simulink model "PMSM_DTC_Traditional_Control"  (R2022b)
settings: Solver=ode23tb  StartTime=0.0  StopTime=0.4  RelTol=1e-4
libraries: spsDCVoltageSourceLib x1, spsGroundLib x1, slpidlib x1, spsPermanentMagnetSynchronousMachineLib x1, spsThreePhaseVIMeasurementLib x1, spsTwoLevelConverterLib x1, spspowerguiLib x1
settings Model: Creator=31904  LastModifiedBy=31904
settings SolverCC: ZeroCrossAlgorithm=Adaptive
settings DebuggingCC: IgnoredZcDiagnostic=none

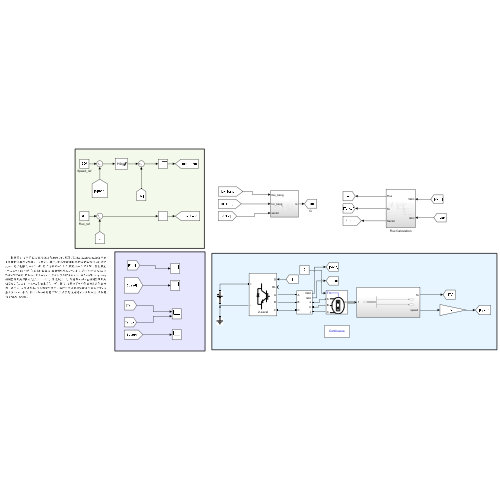
[thumbnail: Simulink's stored preview of the top-level diagram]
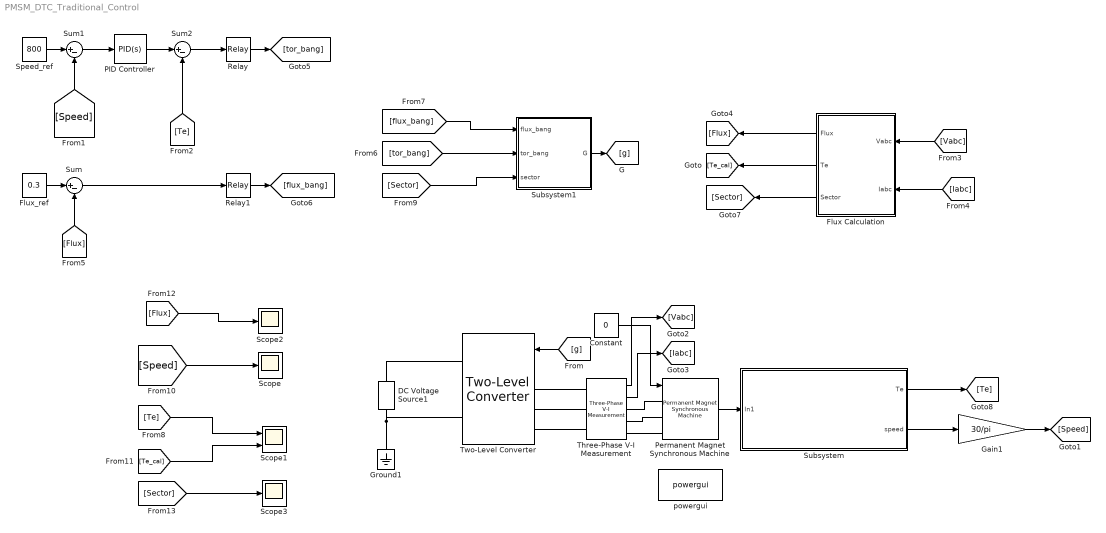
== system PMSM_DTC_Traditional_Control ==
  Constant : Constant  Value=0
  DC Voltage Source1 : spsDCVoltageSourceLib/DC Voltage Source  Amplitude=311  Measurements=None
  Flux Calculation : Subsystem
  Flux_ref : Constant  Value=0.3
  Gain1 : Gain  Gain=30/pi
  Ground1 : spsGroundLib/Ground  LConnTagsString=a
  PID Controller : slpidlib/PID Controller  Controller=PID  Form=Parallel  TimeDomain=Continuous-time  UseExternalTs=off  SampleTime=-1  IntegratorMethod=Forward Euler  FilterMethod=Forward Euler  ControllerParametersSource=internal  P=0.1  I=5  UseKiTs=off  D=0  N=100  UseFilter=on  TunerSelectOption=Transfer Function Based (PID Tuner App)  ZeroCross=off  InitialConditionSource=internal  InitialConditionForIntegrator=0  InitialConditionForFilter=0  DifferentiatorICPrevScaledInput=0  ExternalReset=none  TrackingMode=off  Kt=1  LimitOutput=on  SatLimitsSource=internal  UpperSaturationLimit=5  LowerSaturationLimit=-5  LinearizeAsGain=on  AntiWindupMode=none  Kb=1  LimitIntegrator=off  UpperIntegratorSaturationLimit=inf  LowerIntegratorSaturationLimit=-inf  POutMin=[]  POutMax=[]  IOutMin=[]  IOutMax=[]  DOutMin=[]  DOutMax=[]  NOutMin=[]  NOutMax=[]  SumOutMin=[]  SumOutMax=[]  SaturationOutMin=[]  SaturationOutMax=[]  PParamMin=[]  PParamMax=[]  IParamMin=[]  IParamMax=[]  DParamMin=[]  DParamMax=[]  NParamMin=[]  NParamMax=[]  KbParamMin=[]  KbParamMax=[]  KtParamMin=[]  KtParamMax=[]  KbOutMin=[]  KbOutMax=[]  KtOutMin=[]  KtOutMax=[]  IntegratorOutMin=[]  IntegratorOutMax=[]  FilterOutMin=[]  FilterOutMax=[]  SumI1OutMin=[]  SumI1OutMax=[]  SumI2OutMin=[]  SumI2OutMax=[]  SumI3OutMin=[]  SumI3OutMax=[]  SumI4OutMin=[]  SumI4OutMax=[]  SumDOutMin=[]  SumDOutMax=[]  DifferentiatorOutMin=[]  DifferentiatorOutMax=[]  FilterDiffOutCoefMin=[]  FilterDiffOutCoefMax=[]  ReciprocalOutMin=[]  ReciprocalOutMax=[]  SumDenOutMin=[]  SumDenOutMax=[]  SumNumOutMin=[]  SumNumOutMax=[]  DivideOutMin=[]  DivideOutMax=[]  UdiffTsProdOutMin=[]  UdiffTsProdOutMax=[]  NTsProdOutMin=[]  NTsProdOutMax=[]  UintegralTsProdOutMin=[]  UintegralTsProdOutMax=[]  UngainTsProdOutMin=[]  UngainTsProdOutMax=[]  ClampingZeroOutDataTypeStr=Inherit: Inherit via back propagation  ClampingZeroOutMin=[]  ClampingZeroOutMax=[]  FilterDenConstantOutDataTypeStr=Inherit: Inherit via back propagation  FilterDenConstantOutMin=[]  FilterDenConstantOutMax=[]  PCopyOutDataTypeStr=Inherit: Inherit via back propagation  PCopyOutMin=[]  PCopyOutMax=[]  NCopyOutDataTypeStr=Inherit: Inherit via back propagation  NCopyOutMin=[]  NCopyOutMax=[]  IntegratorContinuousStateAttributes=''  IntegratorStateMustResolveToSignalObject=off  IntegratorRTWStateStorageClass=Auto  FilterContinuousStateAttributes=''  FilterStateMustResolveToSignalObject=off  FilterRTWStateStorageClass=Auto  ParallelPVariant=InternalParameters  IdealPVariant=Disabled  IVariant=InternalParameters  DVariant=InternalParameters  IntegratorVariant=Continuous  SatVariant=Enabled  AWVariant=Passthrough  PCopyVariant=Disabled  TRVariant=Disabled  FdbkBlocksVariant=Forward  IdealPFdbkVariant=Disabled  SatFdbkVariant=Disabled  DerivativeFilterVariant=ContFilter  NVariant=InternalParameters  NCopyVariant=Disabled  FilterICVariant=InternalICsFilter  IntegratorICVariant=InternalICs  ExternalResetVariant=Disabled  TRSumVariant=Passthrough  SumFdbkVariant=Disabled  SumVariant=Sum_PID  TsampFilterVariant=InternalTs  TsampNgainVariant=Passthrough  TsampIntegralVariant=Passthrough  ExternalSaturationOutDataTypeStr=Inherit: Same as second input
  Permanent Magnet Synchronous Machine : spsPermanentMagnetSynchronousMachineLib/Permanent Magnet Synchronous Machine  NbPhases=3  FluxDistribution=Sinusoidal  RotorType=Salient-pole  MechanicalLoad=Torque Tm  PresetModel=No  ShowDetailedParameters=on  MeasurementBus=off  Resistance=1.2  Inductance=8.5e-3  dqInductances=[8.5e-3,8.5e-3]  La=0.0085  MachineConstant=Flux linkage established by magnets (V.s)  Flux=0.175  VoltageCst=126.966  TorqueCst=1.05  Flat=120  Mechanical=[0.0008 0 4 0]  PolePairs=4  InitialConditions=[0,0, 0,0]  InitialConditions5ph=[0 0 0 0 0 0]  RefAngle=90 degrees behind phase A axis (modified Park)  IterativeDiscreteModel=Trapezoidal non iterative  TsBlock=-1  TsPowergui=0
  Relay : Relay  OnSwitchValue=0.1  OffSwitchValue=-0.1
  Relay1 : Relay  OnSwitchValue=0.002  OffSwitchValue=-0.002  ZeroCross=off
  Scope : Scope
  Scope1 : Scope  NumInputPorts=2
  Scope2 : Scope
  Scope3 : Scope
  Speed_ref : Constant  Value=800
  Subsystem : Subsystem
  Subsystem1 : Subsystem
  Sum : Sum  Inputs=|+-
  Sum1 : Sum  Inputs=|+-
  Sum2 : Sum  Inputs=|+-
  Three-Phase V-I Measurement : spsThreePhaseVIMeasurementLib/Three-Phase V-I Measurement  VoltageMeasurement=phase-to-ground  SetLabelV=off  LabelV=Vabc  Vpu=off  VpuLL=off  CurrentMeasurement=yes  SetLabelI=off  LabelI=Iabc  Ipu=off  Pbase=100e6  Vbase=500e3  OutputType=Complex  PhasorSimulation=off  PSBequivalent=0
  Two-Level Converter : spsTwoLevelConverterLib/Two-Level Converter  ModelType=Switching devices  Ron=1e-3  Rs=1e6  Cs=inf  Vforward=[0,0]  Ron_Diode=1e-3  Rs_Diode=1e6  Cs_Diode=inf  Vf_Diode=1e-3  Rs_CurrentSource=inf  Ron_ACsource=1e-3
      settings: LibrarySourceBlock=sps_lib/Power Electronics/Two-Level Converter
  powergui : spspowerguiLib/powergui  Priority=1  SimulationMode=Continuous  SampleTime=50e-6  frequency=60  Iterations=50  frequencyindice=0  Pbase=100e6  ErrMax=1e-4  UnitsV=kV  UnitsW=MW  buscounter=0  FunctionMessages=off  echomessages=off  EnableUseOfTLC=off  CurrentSourceSwitches=off  DisableSnubberDevices=off  DisableRonSwitches=off  DisableVfSwitches=off  DisplayEquations=off  AutomaticDiscreteSolvers=off  SolverType=Tustin/Backward Euler (TBE)  Interpol=off  ExternalGateDelay=off  methode=off  Ts=100  x0status=blocks  SPID=on  SwTol=0  HookPort=off  NonlinearTolerance=1e-4  nMaxIteration=100  ContinueOnMaxIteration=off  RestoreLinks=warning  ResistiveCurrentMeasurement=off  Frange=[0:2:500]  Ylog=off  Xlog=on  ShowGrid=off  save=off  variable=ZData  structure=0  ZoomFFT=off  StartTime=0.0  cycles=1  DisplayStyle=1  fundamental=60  FreqAxis=off  MaxFrequency=1000  frequencyindicesteady=1  RmsSteady=1  display=off
  wires:
  Permanent Magnet Synchronous Machine/1 -> Subsystem/1(In1)
  [g] -> Two-Level Converter/1
  Subsystem/2("speed ") -> Gain1/1
  Three-Phase V-I Measurement/1 -> [Vabc]
  Three-Phase V-I Measurement/2 -> [Iabc]
  [Vabc] -> Flux Calculation/1(Vabc)
  [Iabc] -> Flux Calculation/2(Iabc)
  Flux Calculation/3(Sector) -> [Sector]
  Flux Calculation/1(Flux) -> [Flux]
  [Flux] -> Sum/2
  Flux_ref/1 -> Sum/1
  Speed_ref/1 -> Sum1/1
  [Speed] -> Sum1/2
  Sum1/1 -> PID Controller/1
  PID Controller/1 -> Sum2/1
  [Te] -> Sum2/2
  Gain1/1 -> [Speed]
  Sum2/1 -> Relay/1
  Relay/1 -> [tor_bang]
  Relay1/1 -> [flux_bang]
  Sum/1 -> Relay1/1
  Subsystem1/1(G) -> [g]
  [tor_bang] -> Subsystem1/2(tor_bang)
  [flux_bang] -> Subsystem1/1(flux_bang)
  [Sector] -> Subsystem1/3(sector)
  [Speed] -> Scope/1
  Constant/1 -> Permanent Magnet Synchronous Machine/1
  Subsystem/1(Te) -> [Te]
  [Te] -> Scope1/1
  Flux Calculation/2(Te) -> [Te_cal]
  [Te_cal] -> Scope1/2
  [Flux] -> Scope2/1
  [Sector] -> Scope3/1
  connections:
  Two-Level Converter/RConn1 -- DC Voltage Source1/RConn1
  DC Voltage Source1/LConn1 -- Ground1/LConn1 -- Two-Level Converter/RConn2
  Three-Phase V-I Measurement/LConn1 -- Two-Level Converter/LConn1
  Three-Phase V-I Measurement/LConn2 -- Two-Level Converter/LConn2
  Three-Phase V-I Measurement/LConn3 -- Two-Level Converter/LConn3
  Three-Phase V-I Measurement/RConn1 -- Permanent Magnet Synchronous Machine/LConn1
  Three-Phase V-I Measurement/RConn2 -- Permanent Magnet Synchronous Machine/LConn2
  Three-Phase V-I Measurement/RConn3 -- Permanent Magnet Synchronous Machine/LConn3

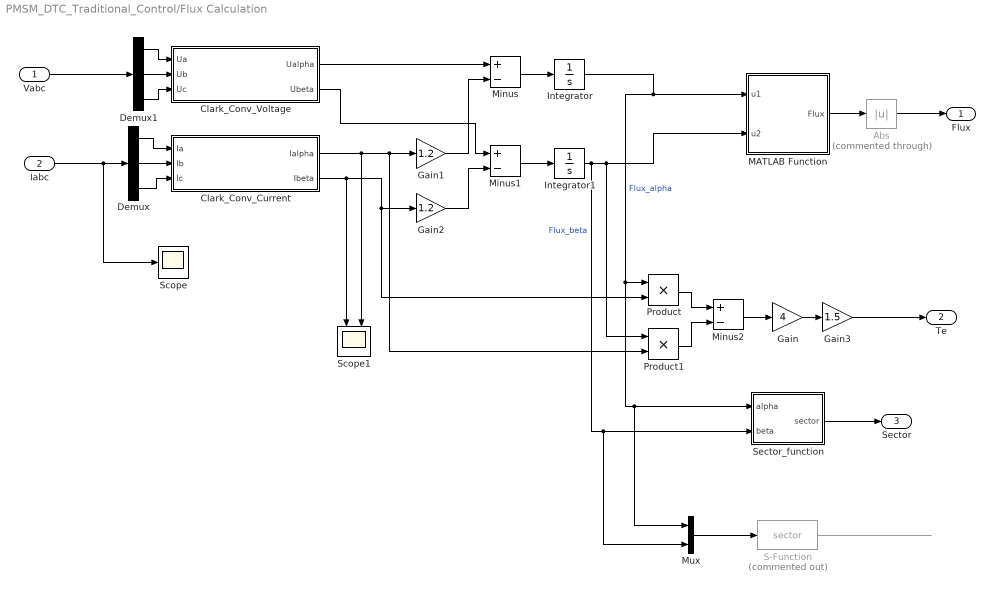
== system PMSM_DTC_Traditional_Control/Flux Calculation ==
  Vabc : Inport
  Iabc : Inport  Port=2
  Abs : Abs  Commented=through  SaturateOnIntegerOverflow=off
  Clark_Conv_Current : Subsystem
  Clark_Conv_Voltage : Subsystem
  Demux : Demux  Outputs=3
  Demux1 : Demux  Outputs=3
  Gain : Gain  Gain=4
  Gain1 : Gain  Gain=1.2
  Gain2 : Gain  Gain=1.2
  Gain3 : Gain  Gain=1.5
  Integrator : Integrator
  Integrator1 : Integrator
  MATLAB Function : MATLAB Function  TreatAsAtomicUnit=on
  Minus : Sum  Inputs=+-
  Minus1 : Sum  Inputs=+-
  Minus2 : Sum  Inputs=+-
  Mux : Mux  Inputs=2
  Product : Product
  Product1 : Product
  S-Function : S-Function  Commented=on  FunctionName=sector  SFunctionDeploymentMode=off  EnableBusSupport=off
  Scope : Scope
  Scope1 : Scope  NumInputPorts=2
  Sector_function : MATLAB Function  TreatAsAtomicUnit=on
  Flux : Outport
  Te : Outport  Port=2
  Sector : Outport  Port=3
  wires:
  Demux/1 -> Clark_Conv_Current/1(Ia)
  Demux1/2 -> Clark_Conv_Voltage/2(Ub)
  Demux/2 -> Clark_Conv_Current/2(Ib)
  Demux/3 -> Clark_Conv_Current/3(Ic)
  Clark_Conv_Voltage/1(Ualpha) -> Minus/1
  Demux1/3 -> Clark_Conv_Voltage/3(Uc)
  Clark_Conv_Voltage/2(Ubeta) -> Minus1/1
  Demux1/1 -> Clark_Conv_Voltage/1(Ua)
  Clark_Conv_Current/1(Ialpha) -> Product1/2, Gain1/1, Scope1/2
  Clark_Conv_Current/2(Ibeta) -> Product/2, Gain2/1, Scope1/1
  Vabc/1 -> Demux1/1
  Iabc/1 -> Scope/1, Demux/1
  Gain1/1 -> Minus/2
  Minus/1 -> Integrator/1
  Integrator/1 -> Mux/1, Sector_function/1(alpha), Product/1, MATLAB Function/1(u1)  "Flux_alpha"
  Gain2/1 -> Minus1/2
  Minus1/1 -> Integrator1/1
  Integrator1/1 -> Mux/2, Sector_function/2(beta), MATLAB Function/2(u2), Product1/1  "Flux_beta"
  MATLAB Function/1(Flux) -> Abs/1
  Gain/1 -> Gain3/1
  Product/1 -> Minus2/1
  Product1/1 -> Minus2/2
  Minus2/1 -> Gain/1
  Gain3/1 -> Te/1
  Abs/1 -> Flux/1
  Mux/1 -> S-Function/1
  S-Function/1 -> ?
  Sector_function/1(sector) -> Sector/1

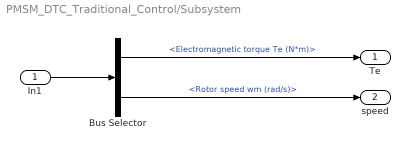
== system PMSM_DTC_Traditional_Control/Subsystem ==
  In1 : Inport
  Bus Selector : BusSelector  OutputSignals=Electromagnetic torque Te (N*m),Rotor speed wm (rad/s)
  Te : Outport
  "speed " : Outport  Port=2
  wires:
  In1/1 -> Bus Selector/1
  Bus Selector/1 -> Te/1  "<Electromagnetic torque Te (N*m)>"
  Bus Selector/2 -> "speed "/1  "<Rotor speed wm (rad/s)>"

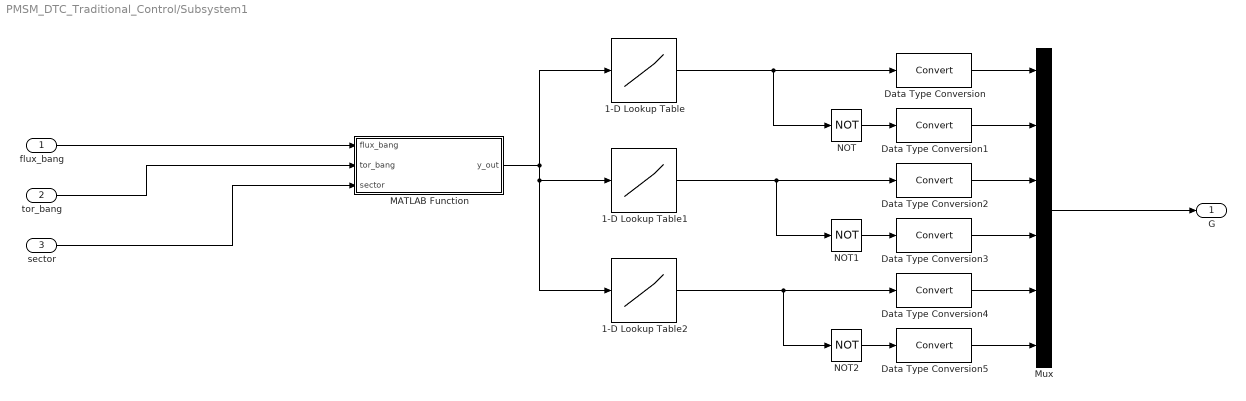
== system PMSM_DTC_Traditional_Control/Subsystem1 ==
  flux_bang : Inport
  tor_bang : Inport  Port=2
  sector : Inport  Port=3
  1-D Lookup Table : Lookup_n-D  NumberOfTableDimensions=1  BreakpointsForDimension1=[1,2,3,4,5,6]  Table=[0 0 0 1 1 1]  InternalRulePriority=Speed  RndMeth=Simplest
  1-D Lookup Table1 : Lookup_n-D  NumberOfTableDimensions=1  BreakpointsForDimension1=[1,2,3,4,5,6]  Table=[0 1 1 0 0 1]  InternalRulePriority=Speed  RndMeth=Simplest
  1-D Lookup Table2 : Lookup_n-D  NumberOfTableDimensions=1  BreakpointsForDimension1=[1,2,3,4,5,6]  Table=[1 0 1 0 1 0]  InternalRulePriority=Speed  RndMeth=Simplest
  Data Type Conversion{,1..5} (6 alike) : DataTypeConversion  SaturateOnIntegerOverflow=off  RndMeth=Floor
  MATLAB Function : MATLAB Function  TreatAsAtomicUnit=on
  Mux : Mux  Inputs=6
  NOT : Logic  Operator=NOT  IconShape=distinctive  AllPortsSameDT=off  OutDataTypeStr=boolean
  NOT1 : Logic  Operator=NOT  IconShape=distinctive  AllPortsSameDT=off  OutDataTypeStr=boolean
  NOT2 : Logic  Operator=NOT  IconShape=distinctive  AllPortsSameDT=off  OutDataTypeStr=boolean
  G : Outport
  wires:
  sector/1 -> MATLAB Function/3(sector)
  tor_bang/1 -> MATLAB Function/2(tor_bang)
  flux_bang/1 -> MATLAB Function/1(flux_bang)
  MATLAB Function/1(y_out) -> 1-D Lookup Table/1, 1-D Lookup Table2/1, 1-D Lookup Table1/1
  1-D Lookup Table2/1 -> NOT2/1, Data Type Conversion4/1
  1-D Lookup Table/1 -> NOT/1, Data Type Conversion/1
  NOT/1 -> Data Type Conversion1/1
  1-D Lookup Table1/1 -> Data Type Conversion2/1, NOT1/1
  NOT1/1 -> Data Type Conversion3/1
  NOT2/1 -> Data Type Conversion5/1
  Mux/1 -> G/1
  Data Type Conversion/1 -> Mux/1
  Data Type Conversion1/1 -> Mux/2
  Data Type Conversion2/1 -> Mux/3
  Data Type Conversion3/1 -> Mux/4
  Data Type Conversion4/1 -> Mux/5
  Data Type Conversion5/1 -> Mux/6

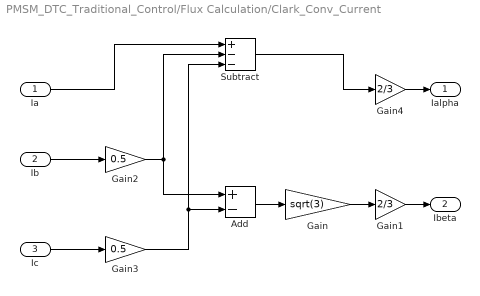
== system PMSM_DTC_Traditional_Control/Flux Calculation/Clark_Conv_Current ==
  Ia : Inport
  Ib : Inport  Port=2
  Ic : Inport  Port=3
  Add : Sum  Inputs=+-
  Gain : Gain  Gain=sqrt(3)
  Gain1 : Gain  Gain=2/3
  Gain2 : Gain  Gain=0.5
  Gain3 : Gain  Gain=0.5
  Gain4 : Gain  Gain=2/3
  Subtract : Sum  Inputs=+--
  Ialpha : Outport
  Ibeta : Outport  Port=2
  wires:
  Ia/1 -> Subtract/1
  Ib/1 -> Gain2/1
  Add/1 -> Gain/1
  Gain/1 -> Gain1/1
  Ic/1 -> Gain3/1
  Gain2/1 -> Subtract/2, Add/1
  Gain3/1 -> Subtract/3, Add/2
  Subtract/1 -> Gain4/1
  Gain4/1 -> Ialpha/1
  Gain1/1 -> Ibeta/1

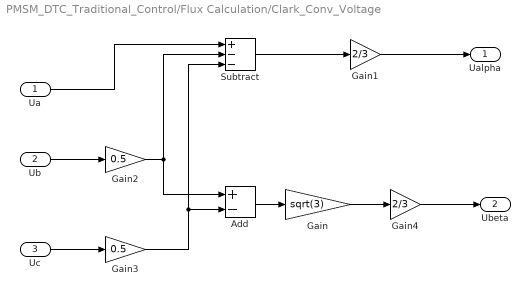
== system PMSM_DTC_Traditional_Control/Flux Calculation/Clark_Conv_Voltage ==
  Ua : Inport
  Ub : Inport  Port=2
  Uc : Inport  Port=3
  Add : Sum  Inputs=+-
  Gain : Gain  Gain=sqrt(3)
  Gain1 : Gain  Gain=2/3
  Gain2 : Gain  Gain=0.5
  Gain3 : Gain  Gain=0.5
  Gain4 : Gain  Gain=2/3
  Subtract : Sum  Inputs=+--
  Ualpha : Outport
  Ubeta : Outport  Port=2
  wires:
  Subtract/1 -> Gain1/1
  Gain3/1 -> Add/2, Subtract/3
  Gain2/1 -> Add/1, Subtract/2
  Uc/1 -> Gain3/1
  Gain/1 -> Gain4/1
  Add/1 -> Gain/1
  Ub/1 -> Gain2/1
  Ua/1 -> Subtract/1
  Gain1/1 -> Ualpha/1
  Gain4/1 -> Ubeta/1

== matlab function PMSM_DTC_Traditional_Control/Flux Calculation/MATLAB Function ==
  data: u1 input; Flux output; u2 input
function Flux = fcn(u1,u2)

Flux = sqrt(u1^2+u2^2);

== matlab function PMSM_DTC_Traditional_Control/Subsystem1/MATLAB Function ==
  data: flux_bang input; tor_bang input; y_out output; sector input
function y_out = fcn(flux_bang,tor_bang,sector)

V_Table=[5 3 1 6 4 2;3 6 2 5 1 4 ;4 1 5 2 6 3;2 4 6 1 3 5];
x=2*flux_bang+tor_bang+1;
y_out=V_Table(x,sector);
end

== matlab function PMSM_DTC_Traditional_Control/Flux Calculation/Sector_function ==
  data: alpha input; sector output; beta input
function sector = fcn(alpha,beta)

if(beta==0)
    sector=1;
else
f1 = alpha;
f2 =-alpha+sqrt(3)*beta;
f3 =-alpha-sqrt(3)*beta;
if(f1>0)
    a=0;
else
    a=1;
end

if(f2>0)
    b=0;
else
    b=1;
end

if(f3>0)
    c=0;
else
    c=1;
end

sector=4*a+2*b+c;
end
